simulink model "wipersubsystem_signal"  (R2020b)
settings: Solver=VariableStepAuto  StartTime=0.0  StopTime=10.0  RelTol=1e-3
undefined symbols (not defined in the file): sigbuilder_block
settings Model: Creator=99003188  LastModifiedBy=99003188

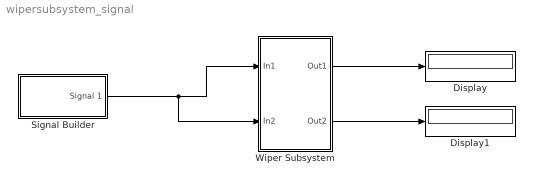
== system wipersubsystem_signal ==
  Display : Display
  Display1 : Display
  Signal Builder : Subsystem  Tag=STV Subsys  LoadFcn=sigbuilder_block('load');  StartFcn=sigbuilder_block('start');  StopFcn=sigbuilder_block('stop');  ClipboardFcn=sigbuilder_block('clipboard');  mask(Sigbuilder block){tuvar=[0:10]}
      mask help: Simulink:masks:SigbuilderBlock_MD
      mask init:
      | if ~strcmp(get_param(bdroot(gcbh),'SimulationStatus'),'stopped') tuvar = sigbuilder_block('maskInit'); end
      settings: CopyFcn=sigbuilder_block('copy');  DeleteFcn=sigbuilder_block('delete');  ModelCloseFcn=sigbuilder_block('modelClose');  PreSaveFcn=sigbuilder_block('preSave');  PauseFcn=sigbuilder_block('pause');  ContinueFcn=sigbuilder_block('continue');  NameChangeFcn=sigbuilder_block('namechange');  OpenFcn=sigbuilder_block('open',[437.6 153 550.4 359.25 ]);  CloseFcn=sigbuilder_block('close');
      mask Display: plot(0, 0, 100, 100,[2, 2, 32, 32, 2], [68, 8, 8, 68, 68],[32, 2], [38, 38], [32, 19, 2],[53, 60, 44], [32, 17, 17, 2],[16, 16, 31, 31]);txt = getActiveGroup(gcbh);text(2, 100, txt,'verticalAlignment', 'top');
  Wiper Subsystem : Subsystem
  wires:
  Wiper Subsystem/2(Out2) -> Display1/1
  Wiper Subsystem/1(Out1) -> Display/1
  Signal Builder/1(Signal 1) -> Wiper Subsystem/2(In2), Wiper Subsystem/1(In1)

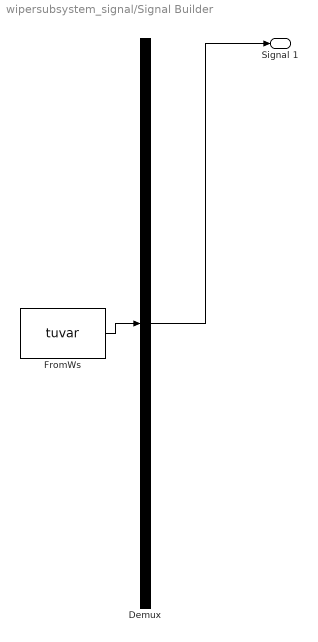
== system wipersubsystem_signal/Signal Builder ==
  Demux : Demux  Tag=STV Demux  Outputs=1
      settings: DisplayOption=none
  FromWs : FromWorkspace  Tag=STV FromWs  VariableName=tuvar
      SigBuilderData=|
      | common.afterFinalStr = 'Extrapolate'
      | common.sampleTime = 0
      | dataSet.timeRange = [0 10]
      | dataSet.name = 'Group 1'
      | sbobj.Groups.Name = 'Group 1'
      | sbobj.Groups.Signals.Name = 'Signal 1'
      | sbobj.Groups.Signals.XData = [0 4 4 6 6 10]
      | sbobj.Groups.Signals.YData = [1 1.03 1.98 1.98 3.02 3.02]
  Signal 1 : Outport  Tag=STV Outport
  wires:
  Demux/1 -> Signal 1/1
  FromWs/1 -> Demux/1

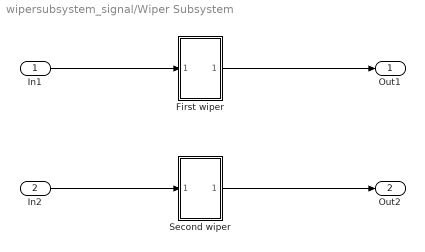
== system wipersubsystem_signal/Wiper Subsystem ==
  In1 : Inport
  In2 : Inport  Port=2
  First wiper : Subsystem
  Second wiper : Subsystem
  Out1 : Outport
  Out2 : Outport  Port=2
  wires:
  In1/1 -> First wiper/1(In1)
  First wiper/1(Out1) -> Out1/1
  Second wiper/1(Out1) -> Out2/1
  In2/1 -> Second wiper/1(In1)

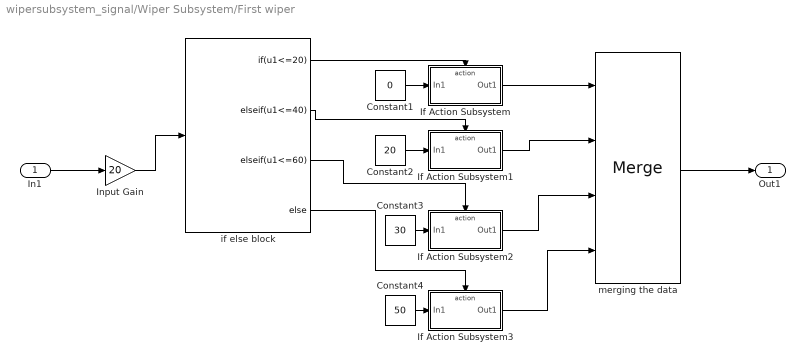
== system wipersubsystem_signal/Wiper Subsystem/First wiper ==
  In1 : Inport
  Constant1 : Constant  Value=0
  Constant2 : Constant  Value=20
  Constant3 : Constant  Value=30
  Constant4 : Constant  Value=50
  If Action Subsystem : Subsystem  TreatAsAtomicUnit=on
  If Action Subsystem1 : Subsystem  TreatAsAtomicUnit=on
  If Action Subsystem2 : Subsystem  TreatAsAtomicUnit=on
  If Action Subsystem3 : Subsystem  TreatAsAtomicUnit=on
  Input Gain : Gain  Gain=20
  if else block : If  IfExpression=u1<=20  ElseIfExpressions=u1<=40,u1<=60
  "merging the data " : Merge  Inputs=4
  Out1 : Outport
  wires:
  if else block/2 -> If Action Subsystem1/Action
  If Action Subsystem3/1(Out1) -> "merging the data "/4
  if else block/1 -> If Action Subsystem/Action
  if else block/3 -> If Action Subsystem2/Action
  Constant4/1 -> If Action Subsystem3/1(In1)
  If Action Subsystem/1(Out1) -> "merging the data "/1
  Constant3/1 -> If Action Subsystem2/1(In1)
  If Action Subsystem1/1(Out1) -> "merging the data "/2
  Input Gain/1 -> if else block/1
  If Action Subsystem2/1(Out1) -> "merging the data "/3
  "merging the data "/1 -> Out1/1
  In1/1 -> Input Gain/1
  Constant2/1 -> If Action Subsystem1/1(In1)
  Constant1/1 -> If Action Subsystem/1(In1)
  if else block/4 -> If Action Subsystem3/Action

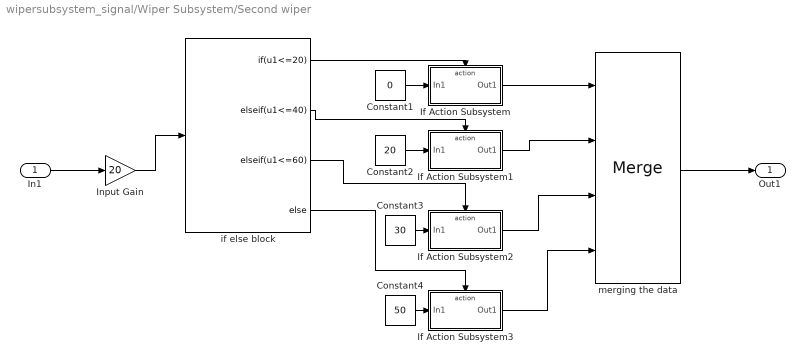
== system wipersubsystem_signal/Wiper Subsystem/Second wiper ==
  In1 : Inport
  Constant1 : Constant  Value=0
  Constant2 : Constant  Value=20
  Constant3 : Constant  Value=30
  Constant4 : Constant  Value=50
  If Action Subsystem : Subsystem  TreatAsAtomicUnit=on
  If Action Subsystem1 : Subsystem  TreatAsAtomicUnit=on
  If Action Subsystem2 : Subsystem  TreatAsAtomicUnit=on
  If Action Subsystem3 : Subsystem  TreatAsAtomicUnit=on
  Input Gain : Gain  Gain=20
  if else block : If  IfExpression=u1<=20  ElseIfExpressions=u1<=40,u1<=60
  "merging the data " : Merge  Inputs=4
  Out1 : Outport
  wires:
  if else block/2 -> If Action Subsystem1/Action
  If Action Subsystem3/1(Out1) -> "merging the data "/4
  if else block/1 -> If Action Subsystem/Action
  if else block/3 -> If Action Subsystem2/Action
  Constant4/1 -> If Action Subsystem3/1(In1)
  If Action Subsystem/1(Out1) -> "merging the data "/1
  Constant3/1 -> If Action Subsystem2/1(In1)
  If Action Subsystem1/1(Out1) -> "merging the data "/2
  Input Gain/1 -> if else block/1
  If Action Subsystem2/1(Out1) -> "merging the data "/3
  "merging the data "/1 -> Out1/1
  In1/1 -> Input Gain/1
  Constant2/1 -> If Action Subsystem1/1(In1)
  Constant1/1 -> If Action Subsystem/1(In1)
  if else block/4 -> If Action Subsystem3/Action

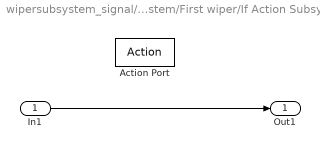
== system wipersubsystem_signal/Wiper Subsystem/First wiper/If Action Subsystem ==
  In1 : Inport
  Action Port : ActionPort  ActionPortLabel=if(u1<=20)
  Out1 : Outport
  wires:
  In1/1 -> Out1/1

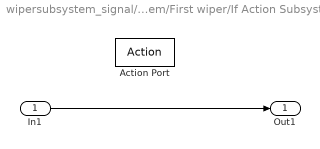
== system wipersubsystem_signal/Wiper Subsystem/First wiper/If Action Subsystem1 ==
  In1 : Inport
  Action Port : ActionPort  ActionPortLabel=elseif(u1<=40)
  Out1 : Outport
  wires:
  In1/1 -> Out1/1

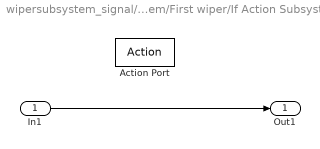
== system wipersubsystem_signal/Wiper Subsystem/First wiper/If Action Subsystem2 ==
  In1 : Inport
  Action Port : ActionPort  ActionPortLabel=elseif(u1<=60)
  Out1 : Outport
  wires:
  In1/1 -> Out1/1

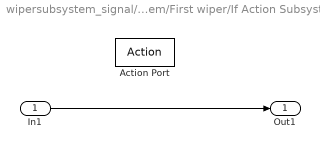
== system wipersubsystem_signal/Wiper Subsystem/First wiper/If Action Subsystem3 ==
  In1 : Inport
  Action Port : ActionPort  ActionPortLabel=else
  Out1 : Outport
  wires:
  In1/1 -> Out1/1

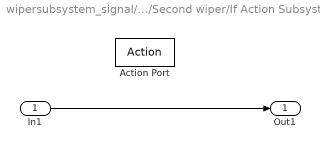
== system wipersubsystem_signal/Wiper Subsystem/Second wiper/If Action Subsystem ==
  In1 : Inport
  Action Port : ActionPort  ActionPortLabel=if(u1<=20)
  Out1 : Outport
  wires:
  In1/1 -> Out1/1

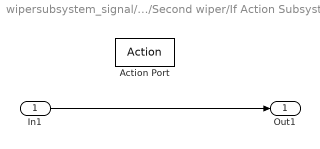
== system wipersubsystem_signal/Wiper Subsystem/Second wiper/If Action Subsystem1 ==
  In1 : Inport
  Action Port : ActionPort  ActionPortLabel=elseif(u1<=40)
  Out1 : Outport
  wires:
  In1/1 -> Out1/1

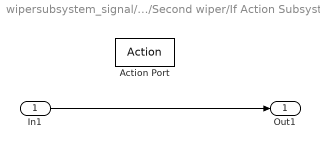
== system wipersubsystem_signal/Wiper Subsystem/Second wiper/If Action Subsystem2 ==
  In1 : Inport
  Action Port : ActionPort  ActionPortLabel=elseif(u1<=60)
  Out1 : Outport
  wires:
  In1/1 -> Out1/1

== system wipersubsystem_signal/Wiper Subsystem/Second wiper/If Action Subsystem3 ==
  In1 : Inport
  Action Port : ActionPort  ActionPortLabel=else
  Out1 : Outport
  wires:
  In1/1 -> Out1/1
